simulink model "wind_speed_model"  (R2024b)
settings: Solver=VariableStepAuto  StartTime=0.0  StopTime=300  RelTol=1e-3
undefined symbols (not defined in the file): dspblkCoreblockFVToolHelper, gcbh
libraries: simulink x2
settings Model: Creator=86189  LastModifiedBy=86189

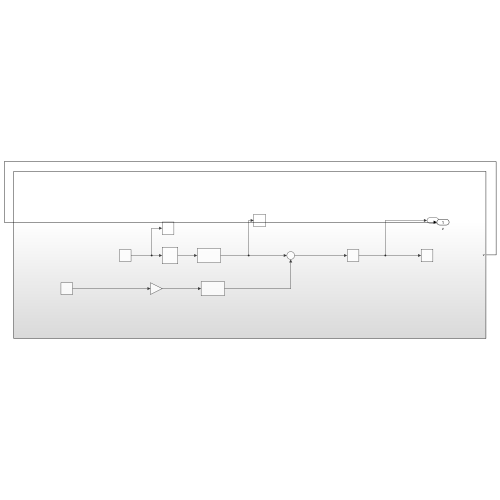
[thumbnail: Simulink's stored preview of the top-level diagram]
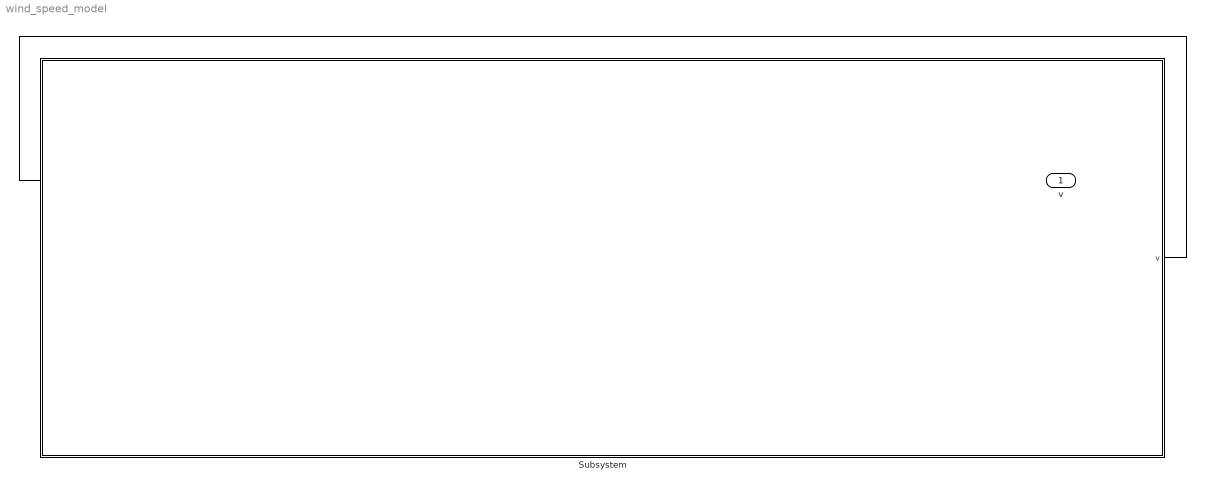
== system wind_speed_model ==
  Subsystem : Subsystem
  v : Outport
  wires:
  Subsystem/1(v) -> v/1

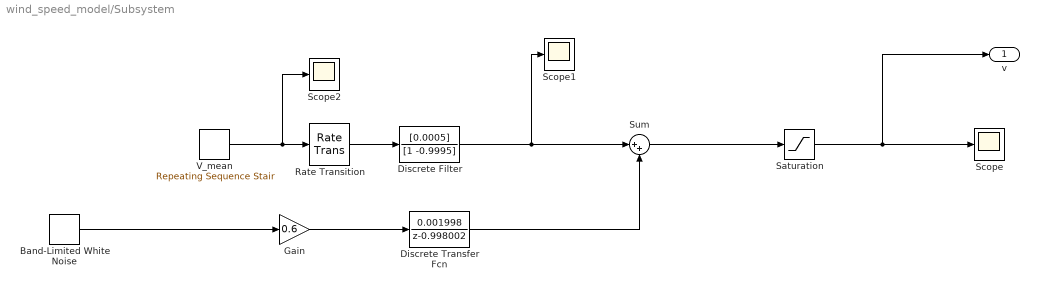
== system wind_speed_model/Subsystem ==
  Band-Limited White Noise : simulink/Sources/Band-Limited White Noise  Cov=[1]  Ts=0.01  seed=[23341]
  Discrete Transfer Fcn : DiscreteTransferFcn  LoadFcn=dspblkCoreblockFVToolHelper(gcbh,'load');  Numerator=[0.001998]  Denominator=[1 -0.998002]
      settings: CopyFcn=dspblkCoreblockFVToolHelper(gcbh,'copy');  DeleteFcn=dspblkCoreblockFVToolHelper(gcbh,'close');  ModelCloseFcn=dspblkCoreblockFVToolHelper(gcbh,'close');  PreSaveFcn=dspblkCoreblockFVToolHelper(gcbh,'presave');  PostSaveFcn=dspblkCoreblockFVToolHelper(gcbh,'postsave');  CloseFcn=dspblkCoreblockFVToolHelper(gcbh,'close');
  Discrete Filter : DiscreteFilter  LoadFcn=dspblkCoreblockFVToolHelper(gcbh,'load');  Numerator=[0.0005]  Denominator=[1 -0.9995]
      settings: CopyFcn=dspblkCoreblockFVToolHelper(gcbh,'copy');  DeleteFcn=dspblkCoreblockFVToolHelper(gcbh,'close');  ModelCloseFcn=dspblkCoreblockFVToolHelper(gcbh,'close');  PreSaveFcn=dspblkCoreblockFVToolHelper(gcbh,'presave');  PostSaveFcn=dspblkCoreblockFVToolHelper(gcbh,'postsave');  CloseFcn=dspblkCoreblockFVToolHelper(gcbh,'close');
  Gain : Gain  Gain=0.6
  Rate Transition : RateTransition  OutPortSampleTime=0.01
  Saturation : Saturate  UpperLimit=25  LowerLimit=0
  Scope : Scope
  Scope1 : Scope
  Scope2 : Scope
  Sum : Sum  Inputs=|++
  V_mean : simulink/Sources/Repeating Sequence Stair  OutValues=[8 6 4 8 12 16 8 14]  tsamp=40  OutMin=[]  OutMax=[]  OutDataTypeStr=double  OutputDataTypeScalingMode=double  OutDataType=fixdt(0,8)  ConRadixGroup=Best Precision: Vector-wise  OutScaling=2^-12
  v : Outport
  wires:
  Discrete Filter/1 -> Scope1/1, Sum/1
  Saturation/1 -> v/1, Scope/1
  Sum/1 -> Saturation/1
  Discrete Transfer Fcn/1 -> Sum/2
  V_mean/1 -> Rate Transition/1, Scope2/1
  Rate Transition/1 -> Discrete Filter/1
  Band-Limited White Noise/1 -> Gain/1
  Gain/1 -> Discrete Transfer Fcn/1
